simulink model "afe_abc_inv_psm_2mods"  (R2025a)
settings: Solver=ode1be  StartTime=0.0  StopTime=simlength  FixedStep=tc  MaxStep=tc
undefined symbols (not defined in the file): Ad_fht, Adrso, afe_pwm_phase_shift_mod1, afe_pwm_phase_shift_mod2, Amplitude_U, Amplitude_V, Amplitude_W, Aresd, b, Bresd, Cfht, Cresd, Crso, CTRPIFF_CLIP_RELEASE, dead_time_AFE, dead_time_INV, deepNEGeta, deepNEGxi, deepPOSxi, emf_fb_p, emf_fb_p_ccaller_1, emf_fb_p_ccaller_2, emf_p, emf_p_ccaller_1, emf_p_ccaller_2, enable_two_modules, end_time_LVRT, fPWM_AFE, fPWM_INV, g0_161Hz, g0_500Hz, g1_161Hz, g1_500Hz, i_grid_neg_eta_lim, i_grid_neg_eta_red_lim, i_grid_neg_xi_lim, i_grid_neg_xi_red_lim, i_grid_pos_eta_lim, i_grid_pos_eta_red_lim, ibez, id_lim, ieta_neg_ref_lim, ieta_pos_ref_lim, Igrid_phase_normalization_factor, inv_pwm_phase_shift_mod1, inv_pwm_phase_shift_mod2, iq_lim, ixi_pos_ref_lim, Jm, k_frt_ref, kg, ki_afe, ki_i, ki_rc_neg_grid, ki_rc_pos_grid, ki_vs, ki_w, kp_afe, kp_i, kp_rc_neg_grid ... (+64)
libraries: spsSampleandHoldLib x213, fl_lib x202, nesl_utility x126, simulink x22, cstblocks x18, threephase_inductor_lib x4, single_phase_transformer_lib x3, flexshaft_lib x1, pmsm_uvw_with_harmonics_lib x1
(part 17 of 18)

== system afe_abc_inv_psm_2mods/afe_abc_inv_psm_mod2/afe_control/grid_voltage_phase_lock_loops/DDSRF-PLL/pll_stageA/mormalization_and_transformation/Subsystem1 ==
  In : Inport
  Sample and Hold : spsSampleandHoldLib/Sample and Hold  ic=0  Ts=0
  Out : Outport
  wires:
  In/1 -> Sample and Hold/1
  [TRGO_afe_module_2] -> Sample and Hold/2
  Sample and Hold/1 -> Out/1

== system afe_abc_inv_psm_2mods/afe_abc_inv_psm_mod2/afe_control/grid_voltage_phase_lock_loops/DDSRF-PLL/pll_stageA/mormalization_and_transformation/Subsystem2 ==
  In : Inport
  Sample and Hold : spsSampleandHoldLib/Sample and Hold  ic=0  Ts=0
  Out : Outport
  wires:
  Sample and Hold/1 -> Out/1
  [TRGO_afe_module_2] -> Sample and Hold/2
  In/1 -> Sample and Hold/1

== system afe_abc_inv_psm_2mods/afe_abc_inv_psm_mod2/afe_control/grid_voltage_phase_lock_loops/DDSRF-PLL/pll_stageA/mormalization_and_transformation/Subsystem5 ==
  In : Inport
  Sample and Hold : spsSampleandHoldLib/Sample and Hold  ic=0  Ts=0
  Out : Outport
  wires:
  In/1 -> Sample and Hold/1
  [TRGO_afe_module_2] -> Sample and Hold/2
  Sample and Hold/1 -> Out/1

== system afe_abc_inv_psm_2mods/afe_abc_inv_psm_mod2/afe_control/grid_voltage_phase_lock_loops/DDSRF-PLL/pll_stageA/sequences/ddsrf ==
  u_grid_alpha : Inport
  u_grid_beta : Inport  Port=2
  phase_angle : Inport  Port=3
  Gain : Gain  Gain=2
  LTI System{,1..3} (4 alike) : cstblocks/LTI System  sys=ddsrf_fd  IC=[]  PadeOrder=0
  Sum : Sum  Inputs=|+-
  Sum1 : Sum  Inputs=|+-
  Sum2 : Sum  Inputs=-+|
  Sum3 : Sum  Inputs=-+|
  alphabeta2xieta_neg : MATLAB Function  TreatAsAtomicUnit=on
  alphabeta2xieta_neg1 : MATLAB Function  TreatAsAtomicUnit=on
  alphabeta2xieta_pos : MATLAB Function  TreatAsAtomicUnit=on
  alphabeta2xieta_pos1 : MATLAB Function  TreatAsAtomicUnit=on
  bounder2 : MATLAB Function  TreatAsAtomicUnit=on  SystemSampleTime=ts_afe
  u_grid_pos_xi : Outport
  u_grid_pos_eta : Outport  Port=2
  u_grid_neg_xi : Outport  Port=3
  u_grid_neg_eta : Outport  Port=4
  wires:
  alphabeta2xieta_neg1/2(eta) -> Sum3/1
  alphabeta2xieta_neg1/1(xi) -> Sum2/1
  alphabeta2xieta_pos1/2(eta) -> Sum1/2
  alphabeta2xieta_pos1/1(xi) -> Sum/2
  [phase_angle_2] -> alphabeta2xieta_neg1/3(gamma)
  [phase_angle_2] -> alphabeta2xieta_pos1/3(gamma)
  bounder2/1(y) -> [phase_angle_2]
  LTI System3/1 -> alphabeta2xieta_pos1/2(beta), u_grid_neg_eta/1
  LTI System2/1 -> alphabeta2xieta_pos1/1(alpha), u_grid_neg_xi/1
  LTI System1/1 -> u_grid_pos_eta/1, alphabeta2xieta_neg1/2(beta)
  LTI System/1 -> u_grid_pos_xi/1, alphabeta2xieta_neg1/1(alpha)
  Gain/1 -> bounder2/1(u)
  alphabeta2xieta_neg/2(eta) -> Sum3/2  "u_grid_neg_eta"
  Sum3/1 -> LTI System3/1
  Sum2/1 -> LTI System2/1
  alphabeta2xieta_neg/1(xi) -> Sum2/2  "u_grid_neg_xi"
  Sum1/1 -> LTI System1/1
  alphabeta2xieta_pos/2(eta) -> Sum1/1  "u_grid_pos_eta"
  Sum/1 -> LTI System/1
  alphabeta2xieta_pos/1(xi) -> Sum/1  "u_grid_pos_xi"
  u_grid_alpha/1 -> alphabeta2xieta_neg/1(alpha), alphabeta2xieta_pos/1(alpha)  "u_grid_alpha"
  u_grid_beta/1 -> alphabeta2xieta_neg/2(beta), alphabeta2xieta_pos/2(beta)  "u_grid_beta"
  phase_angle/1 -> Gain/1, alphabeta2xieta_neg/3(gamma), alphabeta2xieta_pos/3(gamma)  "phase_angle"

== system afe_abc_inv_psm_2mods/afe_abc_inv_psm_mod2/afe_control/grid_voltage_phase_lock_loops/DDSRF-PLL/pll_stageB/double_integrator_observer/Subsystem5 ==
  In : Inport
  Sample and Hold : spsSampleandHoldLib/Sample and Hold  ic=0  Ts=0
  Out : Outport
  wires:
  Sample and Hold/1 -> Out/1
  [TRGO_afe_module_1] -> Sample and Hold/2
  In/1 -> Sample and Hold/1

== system afe_abc_inv_psm_2mods/afe_abc_inv_psm_mod2/afe_control/grid_voltage_phase_lock_loops/DQ-PLL/pll_stageA/mormalization_and_transformation/Subsystem1 ==
  In : Inport
  Sample and Hold : spsSampleandHoldLib/Sample and Hold  ic=0  Ts=0
  Out : Outport
  wires:
  In/1 -> Sample and Hold/1
  [TRGO_afe_module_2] -> Sample and Hold/2
  Sample and Hold/1 -> Out/1

== system afe_abc_inv_psm_2mods/afe_abc_inv_psm_mod2/afe_control/grid_voltage_phase_lock_loops/DQ-PLL/pll_stageA/mormalization_and_transformation/Subsystem2 ==
  In : Inport
  Sample and Hold : spsSampleandHoldLib/Sample and Hold  ic=0  Ts=0
  Out : Outport
  wires:
  Sample and Hold/1 -> Out/1
  [TRGO_afe_module_2] -> Sample and Hold/2
  In/1 -> Sample and Hold/1

== system afe_abc_inv_psm_2mods/afe_abc_inv_psm_mod2/afe_control/grid_voltage_phase_lock_loops/DQ-PLL/pll_stageA/mormalization_and_transformation/Subsystem5 ==
  In : Inport
  Sample and Hold : spsSampleandHoldLib/Sample and Hold  ic=0  Ts=0
  Out : Outport
  wires:
  In/1 -> Sample and Hold/1
  [TRGO_afe_module_2] -> Sample and Hold/2
  Sample and Hold/1 -> Out/1

== system afe_abc_inv_psm_2mods/afe_abc_inv_psm_mod2/afe_control/grid_voltage_phase_lock_loops/DQ-PLL/pll_stageA/mormalization_and_transformation/u_500Hz_flt ==
  input : Inport
  Gain3 : Gain  Gain=g1_500Hz
  Gain6 : Gain  Gain=g0_500Hz
  Sum : Sum  Inputs=|++
  Unit Delay1 : UnitDelay  SampleTime=ts_afe  HasFrameUpgradeWarning=on
  output : Outport  VectorParamsAs1DForOutWhenUnconnected=off
  wires:
  Gain6/1 -> Sum/1
  input/1 -> Gain6/1
  Unit Delay1/1 -> Gain3/1
  Gain3/1 -> Sum/2
  Sum/1 -> Unit Delay1/1, output/1

== system afe_abc_inv_psm_2mods/afe_abc_inv_psm_mod2/afe_control/grid_voltage_phase_lock_loops/DQ-PLL/pll_stageA/mormalization_and_transformation/u_500Hz_flt1 ==
  input : Inport
  Gain3 : Gain  Gain=g1_500Hz
  Gain6 : Gain  Gain=g0_500Hz
  Sum : Sum  Inputs=|++
  Unit Delay1 : UnitDelay  SampleTime=ts_afe  HasFrameUpgradeWarning=on
  output : Outport  VectorParamsAs1DForOutWhenUnconnected=off
  wires:
  Sum/1 -> output/1, Unit Delay1/1
  Gain3/1 -> Sum/2
  Unit Delay1/1 -> Gain3/1
  input/1 -> Gain6/1
  Gain6/1 -> Sum/1

== system afe_abc_inv_psm_2mods/afe_abc_inv_psm_mod2/afe_control/grid_voltage_phase_lock_loops/DQ-PLL/pll_stageA/mormalization_and_transformation/u_500Hz_flt2 ==
  input : Inport
  Gain3 : Gain  Gain=g1_500Hz
  Gain6 : Gain  Gain=g0_500Hz
  Sum : Sum  Inputs=|++
  Unit Delay1 : UnitDelay  SampleTime=ts_afe  HasFrameUpgradeWarning=on
  output : Outport  VectorParamsAs1DForOutWhenUnconnected=off
  wires:
  Gain6/1 -> Sum/1
  input/1 -> Gain6/1
  Unit Delay1/1 -> Gain3/1
  Gain3/1 -> Sum/2
  Sum/1 -> Unit Delay1/1, output/1

== system afe_abc_inv_psm_2mods/afe_abc_inv_psm_mod2/afe_control/grid_voltage_phase_lock_loops/DQ-PLL/pll_stageA/sequences/alphabeta2xieta ==
  alpha : Inport
  beta : Inport  Port=2
  gamma : Inport  Port=3
  alphabeta2xieta_neg : MATLAB Function  TreatAsAtomicUnit=on  SystemSampleTime=ts_afe
  alphabeta2xieta_pos : MATLAB Function  TreatAsAtomicUnit=on  SystemSampleTime=ts_afe
  xi : Outport
  eta : Outport  Port=2
  Out3 : Outport  Port=3
  Out4 : Outport  Port=4
  wires:
  alphabeta2xieta_neg/2(eta) -> Out4/1  "u_grid_neg_eta"
  alphabeta2xieta_neg/1(xi) -> Out3/1  "u_grid_neg_xi"
  alphabeta2xieta_pos/2(eta) -> eta/1  "u_grid_pos_eta"
  alphabeta2xieta_pos/1(xi) -> xi/1  "u_grid_pos_xi"
  gamma/1 -> alphabeta2xieta_pos/3(gamma), alphabeta2xieta_neg/3(gamma)  "gamma_grid"
  beta/1 -> alphabeta2xieta_pos/2(beta), alphabeta2xieta_neg/2(beta)  "u_grid_beta"
  alpha/1 -> alphabeta2xieta_pos/1(alpha), alphabeta2xieta_neg/1(alpha)  "u_grid_alpha"

== system afe_abc_inv_psm_2mods/afe_abc_inv_psm_mod2/afe_control/grid_voltage_phase_lock_loops/DQ-PLL/pll_stageB/double_integrator_observer/Subsystem6 ==
  In : Inport
  Sample and Hold : spsSampleandHoldLib/Sample and Hold  ic=0  Ts=0
  Out : Outport
  wires:
  Sample and Hold/1 -> Out/1
  [TRGO_afe_module_1] -> Sample and Hold/2
  In/1 -> Sample and Hold/1

== system afe_abc_inv_psm_2mods/afe_abc_inv_psm_mod2/inverter_control/current_ctrl/bemf_observer/phase_fault/phase_fault/drop_phase_zerofor_delta_time ==
  theta_pmsm : Inport
  Product : Product
  Step : Step  Time=time_phase_fault  Before=1  After=0  SampleTime=0
  Step1 : Step  Time=time_phase_fault+3e-3  SampleTime=0
  Sum : Sum  Inputs=|++
  theta : Outport
  wires:
  Step/1 -> Sum/1
  Sum/1 -> Product/2
  Product/1 -> theta/1
  Step1/1 -> Sum/2
  theta_pmsm/1 -> Product/1

== system afe_abc_inv_psm_2mods/afe_abc_inv_psm_mod2/inverter_control/current_ctrl/bemf_observer/phase_fault/phase_fault/hold_phase_for_delta_time ==
  theta_pmsm : Inport
  Enabled Subsystem : Subsystem  TreatAsAtomicUnit=on
  Step : Step  Time=time_phase_fault  Before=1  After=0  SampleTime=0
  Step1 : Step  Time=time_phase_fault+25e-3  SampleTime=0
  Sum : Sum  Inputs=|++
  theta : Outport
  wires:
  Sum/1 -> Enabled Subsystem/Enable
  Enabled Subsystem/1(theta) -> theta/1
  theta_pmsm/1 -> Enabled Subsystem/1(theta_pmsm)
  Step1/1 -> Sum/2
  Step/1 -> Sum/1

== system afe_abc_inv_psm_2mods/afe_abc_inv_psm_mod2/inverter_control/current_ctrl/bemf_observer/phase_fault/phase_fault/loss_phase ==
  theta_pmsm : Inport
  Enabled Subsystem : Subsystem  TreatAsAtomicUnit=on
  Step : Step  Time=time_phase_fault  Before=1  After=0  SampleTime=0
  theta : Outport
  wires:
  theta_pmsm/1 -> Enabled Subsystem/1(theta_pmsm)
  Enabled Subsystem/1(theta) -> theta/1
  Step/1 -> Enabled Subsystem/Enable

== system afe_abc_inv_psm_2mods/afe_abc_inv_psm_mod2/inverter_control/current_ctrl/current_ctrl/dq_pi_with_vector_antiwindup/dq_vector_pi/bounder1 ==
  md : Inport
  m_1 : Inport  Port=2
  m : Inport  Port=3
  Constant : Constant
  Constant1 : Constant  Value=0
  Divide : Product
  Switch : Switch  Threshold=1  SaturateOnIntegerOverflow=off  InputSameDT=off
  Switch1 : Switch  Threshold=1  SaturateOnIntegerOverflow=off  InputSameDT=off
  md_sat : Outport  VectorParamsAs1DForOutWhenUnconnected=off
  clip : Outport  Port=2  VectorParamsAs1DForOutWhenUnconnected=off
  wires:
  Constant1/1 -> Switch/3
  Constant/1 -> Switch/1
  m/1 -> Switch/2, Switch1/2
  Switch/1 -> clip/1
  Switch1/1 -> md_sat/1
  Divide/1 -> Switch1/1
  m_1/1 -> Divide/1
  md/1 -> Divide/2, Switch1/3

== system afe_abc_inv_psm_2mods/afe_abc_inv_psm_mod2/inverter_control/current_ctrl/current_ctrl/dq_pi_with_vector_antiwindup/dq_vector_pi/bounder2 ==
  m : Inport
  m_1 : Inport  Port=2
  mq : Inport  Port=3
  Constant : Constant
  Constant1 : Constant  Value=0
  Divide : Product
  Switch : Switch  Threshold=1  SaturateOnIntegerOverflow=off  InputSameDT=off
  Switch1 : Switch  Threshold=1  SaturateOnIntegerOverflow=off  InputSameDT=off
  mq_sat : Outport  VectorParamsAs1DForOutWhenUnconnected=off
  clip : Outport  Port=2  VectorParamsAs1DForOutWhenUnconnected=off
  wires:
  mq/1 -> Switch1/3, Divide/2
  m_1/1 -> Divide/1
  Divide/1 -> Switch1/1
  Switch1/1 -> mq_sat/1
  Switch/1 -> clip/1
  m/1 -> Switch/2, Switch1/2
  Constant/1 -> Switch/1
  Constant1/1 -> Switch/3

== system afe_abc_inv_psm_2mods/afe_abc_inv_psm_mod2/inverter_control/current_ctrl/current_ctrl/dq_pi_with_vector_antiwindup/dq_vector_pi/pi_d ==
  id_tilde : Inport
  clip : Inport  Port=2
  1/Ti : Gain  Gain=kp_i  SaturateOnIntegerOverflow=on  OutDataTypeStr=Inherit: Same as input  ParamDataTypeStr=Inherit: Same as input
  Constant : Constant  Value=0
  Sum2 : Sum  Inputs=+-  SaturateOnIntegerOverflow=on
  Sum4 : Sum  SaturateOnIntegerOverflow=on
  Sum5 : Sum  SaturateOnIntegerOverflow=on
  Switch1 : Switch  Threshold=0.5  SaturateOnIntegerOverflow=off  InputSameDT=off
  Switch2 : Switch  Threshold=0.5  SaturateOnIntegerOverflow=off  InputSameDT=off
  Unit Delay1 : UnitDelay  SampleTime=ts_inv  HasFrameUpgradeWarning=on
  Unit Delay2 : UnitDelay  SampleTime=ts_inv  HasFrameUpgradeWarning=on
  kp1 : Gain  Gain=CTRPIFF_CLIP_RELEASE*ts_inv  SaturateOnIntegerOverflow=on  OutDataTypeStr=Inherit: Same as input  ParamDataTypeStr=Inherit: Same as input
  kp2 : Gain  Gain=ki_i*ts_inv  SaturateOnIntegerOverflow=on  OutDataTypeStr=Inherit: Same as input  ParamDataTypeStr=Inherit: Same as input
  ud_out : Outport  VectorParamsAs1DForOutWhenUnconnected=off
  wires:
  Unit Delay1/1 -> [clip]
  Constant/1 -> Switch2/1
  [clip] -> Switch1/2
  [clip] -> Switch2/2
  clip/1 -> Unit Delay1/1
  kp2/1 -> Switch2/3
  Switch2/1 -> Sum4/1
  1/Ti/1 -> Sum5/1
  Unit Delay2/1 -> Sum2/1, kp1/1, Sum4/2
  Sum2/1 -> Switch1/1
  kp1/1 -> Sum2/2
  Sum4/1 -> Switch1/3, Sum5/2
  Switch1/1 -> Unit Delay2/1
  Sum5/1 -> ud_out/1
  id_tilde/1 -> kp2/1, 1/Ti/1

== system afe_abc_inv_psm_2mods/afe_abc_inv_psm_mod2/inverter_control/current_ctrl/current_ctrl/dq_pi_with_vector_antiwindup/dq_vector_pi/pi_q ==
  iq_tilde : Inport
  clip : Inport  Port=2
  1/Ti : Gain  Gain=kp_i  SaturateOnIntegerOverflow=on  OutDataTypeStr=Inherit: Same as input  ParamDataTypeStr=Inherit: Same as input
  Constant : Constant  Value=0
  Sum2 : Sum  Inputs=+-  SaturateOnIntegerOverflow=on
  Sum4 : Sum  SaturateOnIntegerOverflow=on
  Sum5 : Sum  SaturateOnIntegerOverflow=on
  Switch1 : Switch  Threshold=0.5  SaturateOnIntegerOverflow=off  InputSameDT=off
  Switch2 : Switch  Threshold=0.5  SaturateOnIntegerOverflow=off  InputSameDT=off
  Unit Delay1 : UnitDelay  SampleTime=ts_inv  HasFrameUpgradeWarning=on
  Unit Delay2 : UnitDelay  SampleTime=ts_inv  HasFrameUpgradeWarning=on
  kp1 : Gain  Gain=CTRPIFF_CLIP_RELEASE*ts_inv  SaturateOnIntegerOverflow=on  OutDataTypeStr=Inherit: Same as input  ParamDataTypeStr=Inherit: Same as input
  kp2 : Gain  Gain=ki_i*ts_inv  SaturateOnIntegerOverflow=on  OutDataTypeStr=Inherit: Same as input  ParamDataTypeStr=Inherit: Same as input
  Vqs_out : Outport  VectorParamsAs1DForOutWhenUnconnected=off
  wires:
  Sum5/1 -> Vqs_out/1
  Unit Delay1/1 -> [clip]
  iq_tilde/1 -> kp2/1, 1/Ti/1
  Switch1/1 -> Unit Delay2/1
  Sum4/1 -> Switch1/3, Sum5/2
  kp1/1 -> Sum2/2
  Sum2/1 -> Switch1/1
  Unit Delay2/1 -> Sum4/2, kp1/1, Sum2/1
  1/Ti/1 -> Sum5/1
  Switch2/1 -> Sum4/1
  kp2/1 -> Switch2/3
  clip/1 -> Unit Delay1/1
  [clip] -> Switch2/2
  [clip] -> Switch1/2
  Constant/1 -> Switch2/1

== system afe_abc_inv_psm_2mods/afe_abc_inv_psm_mod2/inverter_control/current_ctrl/current_ctrl/dq_pi_with_vector_antiwindup/dq_vector_pi/switch ==
  clip 1 : Inport
  clip 2 : Inport  Port=2
  Constant4 : Constant
  Constant5 : Constant  Value=0
  Sum1 : Sum  SaturateOnIntegerOverflow=on
  Switch : Switch  Threshold=0.5  SaturateOnIntegerOverflow=off  InputSameDT=off
  clip : Outport  VectorParamsAs1DForOutWhenUnconnected=off
  wires:
  clip 2/1 -> Sum1/2
  clip 1/1 -> Sum1/1
  Sum1/1 -> Switch/2
  Constant4/1 -> Switch/1
  Switch/1 -> clip/1
  Constant5/1 -> Switch/3

== system afe_abc_inv_psm_2mods/afe_abc_inv_psm_mod2/inverter_control/current_ctrl/current_ctrl/dq_pi_with_vector_antiwindup/dq_vector_pi/vector lenght ==
  md : Inport
  mq : Inport  Port=2
  Math Function : Math  Operator=magnitude^2  SignedPower=on
  Math Function1 : Math  Operator=magnitude^2  SignedPower=on
  Math Function2 : Math  Operator=reciprocal  SignedPower=on
  Sqrt : Sqrt
  Sum5 : Sum  SaturateOnIntegerOverflow=on
  m_1 : Outport  VectorParamsAs1DForOutWhenUnconnected=off
  m : Outport  Port=2  VectorParamsAs1DForOutWhenUnconnected=off
  wires:
  md/1 -> Math Function/1
  Math Function2/1 -> m_1/1
  Sum5/1 -> Sqrt/1
  Math Function/1 -> Sum5/1
  Math Function1/1 -> Sum5/2
  mq/1 -> Math Function1/1
  Sqrt/1 -> Math Function2/1, m/1

== system afe_abc_inv_psm_2mods/afe_abc_inv_psm_mod2/inverter_control/current_ctrl/current_ctrl/dq_pi_with_vector_antiwindup/dq_vector_pi_ccaller/Reset ==
  Step : Step  Time=0.05  Before=1  After=0  SampleTime=0
  en : Outport
  wires:
  Step/1 -> en/1

== system afe_abc_inv_psm_2mods/afe_abc_inv_psm_mod2/inverter_control/current_ctrl/current_ctrl/dq_pi_with_vector_antiwindup/dq_vector_pi_ccaller/Subsystem1 ==
  In : Inport
  Sample and Hold : spsSampleandHoldLib/Sample and Hold  ic=0  Ts=0
  Out : Outport
  wires:
  Sample and Hold/1 -> Out/1
  [TRGO_inv_module_2] -> Sample and Hold/2
  In/1 -> Sample and Hold/1

== system afe_abc_inv_psm_2mods/afe_abc_inv_psm_mod2/inverter_control/current_ctrl/current_ctrl/dq_pi_with_vector_antiwindup/dq_vector_pi_ccaller/Subsystem10 ==
  In : Inport
  Sample and Hold : spsSampleandHoldLib/Sample and Hold  ic=0  Ts=0
  Out : Outport
  wires:
  In/1 -> Sample and Hold/1
  [TRGO_inv_module_2] -> Sample and Hold/2
  Sample and Hold/1 -> Out/1

== system afe_abc_inv_psm_2mods/afe_abc_inv_psm_mod2/inverter_control/current_ctrl/current_ctrl/dq_pi_with_vector_antiwindup/dq_vector_pi_ccaller/Subsystem11 ==
  In : Inport
  Sample and Hold : spsSampleandHoldLib/Sample and Hold  ic=0  Ts=0
  Out : Outport
  wires:
  Sample and Hold/1 -> Out/1
  [TRGO_inv_module_2] -> Sample and Hold/2
  In/1 -> Sample and Hold/1

== system afe_abc_inv_psm_2mods/afe_abc_inv_psm_mod2/inverter_control/current_ctrl/current_ctrl/dq_pi_with_vector_antiwindup/dq_vector_pi_ccaller/Subsystem2 ==
  In : Inport
  Sample and Hold : spsSampleandHoldLib/Sample and Hold  ic=0  Ts=0
  Out : Outport
  wires:
  In/1 -> Sample and Hold/1
  [TRGO_inv_module_2] -> Sample and Hold/2
  Sample and Hold/1 -> Out/1

== system afe_abc_inv_psm_2mods/afe_abc_inv_psm_mod2/inverter_control/current_ctrl/current_ctrl/dq_pi_with_vector_antiwindup/dq_vector_pi_ccaller/Subsystem23 ==
  In : Inport
  Sample and Hold : spsSampleandHoldLib/Sample and Hold  ic=0  Ts=0
  Out : Outport
  wires:
  In/1 -> Sample and Hold/1
  [TRGO_inv_module_2] -> Sample and Hold/2
  Sample and Hold/1 -> Out/1

== system afe_abc_inv_psm_2mods/afe_abc_inv_psm_mod2/inverter_control/current_ctrl/current_ctrl/dq_pi_with_vector_antiwindup/dq_vector_pi_ccaller/Subsystem3 ==
  In : Inport
  Sample and Hold : spsSampleandHoldLib/Sample and Hold  ic=0  Ts=0
  Out : Outport
  wires:
  Sample and Hold/1 -> Out/1
  [TRGO_inv_module_2] -> Sample and Hold/2
  In/1 -> Sample and Hold/1

== system afe_abc_inv_psm_2mods/afe_abc_inv_psm_mod2/inverter_control/current_ctrl/current_ctrl/dq_pi_with_vector_antiwindup/dq_vector_pi_ccaller/Subsystem4 ==
  In : Inport
  Sample and Hold : spsSampleandHoldLib/Sample and Hold  ic=0  Ts=0
  Out : Outport
  wires:
  In/1 -> Sample and Hold/1
  [TRGO_inv_module_2] -> Sample and Hold/2
  Sample and Hold/1 -> Out/1

== system afe_abc_inv_psm_2mods/afe_abc_inv_psm_mod2/inverter_control/current_ctrl/current_ctrl/dq_pi_with_vector_antiwindup/dq_vector_pi_ccaller/Subsystem5 ==
  In : Inport
  Sample and Hold : spsSampleandHoldLib/Sample and Hold  ic=0  Ts=0
  Out : Outport
  wires:
  Sample and Hold/1 -> Out/1
  [TRGO_inv_module_2] -> Sample and Hold/2
  In/1 -> Sample and Hold/1

== system afe_abc_inv_psm_2mods/afe_abc_inv_psm_mod2/inverter_control/current_ctrl/current_ctrl/dq_pi_with_vector_antiwindup/dq_vector_pi_ccaller/Subsystem6 ==
  In : Inport
  Sample and Hold : spsSampleandHoldLib/Sample and Hold  ic=0  Ts=0
  Out : Outport
  wires:
  In/1 -> Sample and Hold/1
  [TRGO_inv_module_2] -> Sample and Hold/2
  Sample and Hold/1 -> Out/1

== system afe_abc_inv_psm_2mods/afe_abc_inv_psm_mod2/inverter_control/current_ctrl/current_ctrl/dq_pi_with_vector_antiwindup/dq_vector_pi_ccaller/Subsystem7 ==
  In : Inport
  Sample and Hold : spsSampleandHoldLib/Sample and Hold  ic=0  Ts=0
  Out : Outport
  wires:
  Sample and Hold/1 -> Out/1
  [TRGO_inv_module_2] -> Sample and Hold/2
  In/1 -> Sample and Hold/1

== system afe_abc_inv_psm_2mods/afe_abc_inv_psm_mod2/inverter_control/current_ctrl/current_ctrl/dq_pi_with_vector_antiwindup/dq_vector_pi_ccaller/Subsystem8 ==
  In : Inport
  Sample and Hold : spsSampleandHoldLib/Sample and Hold  ic=0  Ts=0
  Out : Outport
  wires:
  In/1 -> Sample and Hold/1
  [TRGO_inv_module_2] -> Sample and Hold/2
  Sample and Hold/1 -> Out/1

== system afe_abc_inv_psm_2mods/afe_abc_inv_psm_mod2/inverter_control/current_ctrl/current_ctrl/dq_pi_with_vector_antiwindup/dq_vector_pi_ccaller/Subsystem9 ==
  In : Inport
  Sample and Hold : spsSampleandHoldLib/Sample and Hold  ic=0  Ts=0
  Out : Outport
  wires:
  Sample and Hold/1 -> Out/1
  [TRGO_inv_module_2] -> Sample and Hold/2
  In/1 -> Sample and Hold/1

== system afe_abc_inv_psm_2mods/afe_abc_inv_psm_mod1/inverter_control/current_ctrl/bemf_observer/phase_fault/phase_fault/hold_phase_for_delta_time/Enabled Subsystem ==
  theta_pmsm : Inport
  Enable : EnablePort
  theta : Outport
  wires:
  theta_pmsm/1 -> theta/1

== system afe_abc_inv_psm_2mods/afe_abc_inv_psm_mod1/inverter_control/current_ctrl/bemf_observer/phase_fault/phase_fault/loss_phase/Enabled Subsystem ==
  theta_pmsm : Inport
  Enable : EnablePort
  theta : Outport
  wires:
  theta_pmsm/1 -> theta/1

== system afe_abc_inv_psm_2mods/afe_abc_inv_psm_mod2/inverter_control/current_ctrl/bemf_observer/phase_fault/phase_fault/hold_phase_for_delta_time/Enabled Subsystem ==
  theta_pmsm : Inport
  Enable : EnablePort
  theta : Outport
  wires:
  theta_pmsm/1 -> theta/1

== system afe_abc_inv_psm_2mods/afe_abc_inv_psm_mod2/inverter_control/current_ctrl/bemf_observer/phase_fault/phase_fault/loss_phase/Enabled Subsystem ==
  theta_pmsm : Inport
  Enable : EnablePort
  theta : Outport
  wires:
  theta_pmsm/1 -> theta/1

== matlab function afe_abc_inv_psm_2mods/afe_abc_inv_psm_mod1/afe_control/current_ctrl/current_transformation/alphabeta2xieta ==
  data: alpha input; xi output; beta input; gamma input; eta output
function [xi,eta] = alphabeta2xieta(alpha,beta,gamma)

    xi  =  alpha*cos(gamma) + beta*sin(gamma);
    eta = -alpha*sin(gamma) + beta*cos(gamma);

end

== matlab function afe_abc_inv_psm_2mods/grid/grid_emulator/grid_emulator/voltage_reference/xieta2alphabeta_pos ==
  data: xi input; alpha output; eta input; gamma input; beta output
function [alpha,beta] = xieta2alphabeta_pos(xi,eta,gamma)

    alpha  =  xi*cos(gamma) - eta*sin(gamma);
    beta = xi*sin(gamma) + eta*cos(gamma);

end

== matlab function afe_abc_inv_psm_2mods/afe_abc_inv_psm_mod1/inverter_control/current_ctrl/current_transformation/uvw2alphabeta ==
  data: u input; alpha output; v input; w input; beta output
function [alpha,beta] = uvw2alphabeta(u,v,w)

alpha = 2/3*(u - 1/2*v - 1/2*w);
beta  = 2/3*(sqrt(3)/2*(v - w));

end

== matlab function afe_abc_inv_psm_2mods/afe_abc_inv_psm_mod1/inverter_control/current_ctrl/dq2alphabeta ==
  data: d input; alpha output; q input; gamma input; beta output
function [alpha,beta] = dq2alphabeta(d,q,gamma)

    alpha  =  d*cos(gamma) - q*sin(gamma);
    beta = d*sin(gamma) + q*cos(gamma);

end

== matlab function afe_abc_inv_psm_2mods/afe_abc_inv_psm_mod1/afe_control/FRT-VDE4110/FRT-Detection/LVRT_detector ==
  data: vxi_p input; vxi_n input; veta_n input; vxi_p_dot input; vxi_n_dot input; enable input; red_dyn_enabled input; pwr_lim_enable output; frt_exceeded output; reset input; frt_active output; frt_state output; red_dyn_active output
function [pwr_lim_enable, frt_exceeded, frt_active, frt_state, red_dyn_active]  = lvrt_detector(vxi_p,vxi_n,veta_n,vxi_p_dot,vxi_n_dot, enable, red_dyn_enabled, reset)

    persistent state count count2 state_pwr_lim
    
    LVRT_IDLE = 0;
    LVRT_ACTIVE = 1;
    LVRT_EXCEEDED = 2;
    
    PWR_LIM_DISABLED = 0;
    PWR_LIM_ENABLED  = 1;
    
    LVRT_VPOS_TH_LOW			= 0.85;
    LVRT_VPOS_TH_HIGH			= 1.15;
    LVRT_SEQ_DETECTION_HYST		= 0.1;
    LVRT_VNEG_TH				= 0.1;
    LVRT_VPOS_DOT_TH			= 3.0;
    LVRT_VNEG_DOT_TH			= 3.0;
    LVRT_VPOS_PWRLIM_TH			= 0.8;
    LVRT_VNEG_PWRLIM_TH			= 0.1;
    LVRT_PWRLIM_HYST			= 0.1;
    LVRT_VPOS_RED_DYN_TH        = 0.7;
    LVRT_VNEG_RED_DYN_TH        = 0.2;
    LVRT_TIME_HOLD_MAX          = 61000;
    
    RED_DYN_NOT_ACTIVE = 0;
    RED_DYN_ACTIVE     = 1;
        
    if isempty(state)
        state = LVRT_IDLE;
        state_pwr_lim = PWR_LIM_DISABLED;
        count = 0;
        count2 = 0;
    end

    vn = sqrt(vxi_n^2+veta_n^2);

    if enable == 1
        
        switch state
            
            case LVRT_IDLE
                if ((vxi_p > LVRT_VPOS_TH_HIGH || vxi_p < LVRT_VPOS_TH_LOW || vn > LVRT_VNEG_TH) ...
                     && (vxi_p_dot > LVRT_VPOS_DOT_TH || vxi_n_dot > LVRT_VNEG_DOT_TH) && ...
                     count2 > 1000)
                    state = LVRT_ACTIVE;
                end
                frt_active = 0;
                frt_exceeded = 0;
                count = 0;
                frt_state = LVRT_IDLE;
                state_pwr_lim = PWR_LIM_DISABLED;                  
                red_dyn_active = RED_DYN_NOT_ACTIVE;
                count2 = count2 + 1;

            case LVRT_ACTIVE
                count2 = 0;
                % LVRT condition not active anymore
                if (vxi_p >= LVRT_VPOS_TH_LOW  + LVRT_SEQ_DETECTION_HYST && ...
                    vxi_p <  LVRT_VPOS_TH_HIGH - LVRT_SEQ_DETECTION_HYST)
                    state = LVRT_IDLE;
                % LVRT exceeded
                elseif (count >= LVRT_TIME_HOLD_MAX)
                    state = LVRT_EXCEEDED;
                end
                
                % handle power limitation
                if (vxi_p < LVRT_VPOS_PWRLIM_TH || vn > LVRT_VNEG_PWRLIM_TH) 
                    state_pwr_lim = PWR_LIM_ENABLED;
                elseif (vxi_p > LVRT_VPOS_PWRLIM_TH + LVRT_PWRLIM_HYST && vn < LVRT_VPOS_PWRLIM_TH - LVRT_PWRLIM_HYST)
                    state_pwr_lim = PWR_LIM_DISABLED;                  
                end
                
                % handle reduced dynamic grid support
                if red_dyn_enabled && (vxi_p < LVRT_VPOS_RED_DYN_TH || vn > LVRT_VNEG_RED_DYN_TH)
                    red_dyn_active = RED_DYN_ACTIVE;
                else
                    red_dyn_active = RED_DYN_NOT_ACTIVE;
                end
                 
                frt_active = 1;
                frt_exceeded = 0;
                frt_state = LVRT_ACTIVE;
                
                count = count + 1;
            
            case LVRT_EXCEEDED

                if ((reset == 1) || (enable == 0))
                    state = LVRT_IDLE;
                else
                    state = LVRT_EXCEEDED;
                end
                
                frt_exceeded = 1;
                frt_active = 0; 
                frt_state = LVRT_EXCEEDED;
                red_dyn_active = RED_DYN_NOT_ACTIVE;
            
            otherwise
                state = LVRT_IDLE;
                frt_active = 0;
                frt_exceeded = 0;
                frt_state = LVRT_IDLE;
                red_dyn_active = RED_DYN_NOT_ACTIVE;
        end
        
        if state_pwr_lim == PWR_LIM_ENABLED
            pwr_lim_enable = 1;
        else
            pwr_lim_enable = 0;
        end      
    else
        state = LVRT_IDLE;
        frt_active = 0;
        pwr_lim_enable = 0;
        frt_exceeded = 0;
        frt_state = LVRT_IDLE;
        red_dyn_active = RED_DYN_NOT_ACTIVE;
    end
end

== matlab function afe_abc_inv_psm_2mods/afe_abc_inv_psm_mod1/brake/MATLAB Function ==
  data: u input; y output; udc_ref input
function y = fcn(u,udc_ref)

persistent enable_brake

udc_brake_min = 1.15;
udc_brake_max = 1.175;

if isempty(enable_brake)
    enable_brake = 0
end

if u >= udc_ref*udc_brake_max
    y = 15;
    enable_brake = 1;
elseif (u < udc_ref*udc_brake_max && u >= udc_ref*udc_brake_min && enable_brake == 1)
    y = 15;
    enable_brake = 1;
elseif (u < udc_ref*udc_brake_max && u >= udc_ref*udc_brake_min && enable_brake == 0)
    y = 0;
    enable_brake = 0;
else
    y = 0;
    enable_brake = 0;
end

% function y = fcn(u,udc_ref)
% 
% persistent enable_brake
% 
% udc_brake_min = 1.145;
% udc_brake_max = 1.165;
% 
% if isempty(enable_brake)
%     enable_brake = 0
% end
% 
% if u >= udc_ref*udc_brake_max
%     y = 15;
%     enable_brake = 1;
% elseif (u < udc_ref*udc_brake_max && u >= udc_ref*udc_brake_min && enable_brake == 1)
%     y = 15;
%     enable_brake = 1;
% elseif (u < udc_ref*udc_brake_max && u >= udc_ref*udc_brake_min && enable_brake == 0)
%     y = 0;
%     enable_brake = 0;
% else
%     y = 0;
%     enable_brake = 0;
end

== matlab function afe_abc_inv_psm_2mods/afe_abc_inv_psm_mod1/inverter/inverter/sv_pwm/modulator1/PWM generator 2/MATLAB Function ==
  data: t input; y output; phase input; period input
function y = trgo(t,phase,period)
x = sin(2*pi/period*t - phase -pi/2);
y = asin(x);

== matlab function afe_abc_inv_psm_2mods/afe_abc_inv_psm_mod1/afe/sv_pwm/modulator1/PWM generator 3/MATLAB Function ==
  data: t input; y output; phase input; period input
function y = trgo(t,phase,period)
x = sin(2*pi/period*t - phase -pi/2);
y = asin(x);

== matlab function afe_abc_inv_psm_2mods/afe_abc_inv_psm_mod1/inverter_control/current_ctrl/bemf_observer/phase_fault/double_integrator_observer/bounder2 ==
  data: u input; y output
function y = bounder(u)
    
    u = -pi + mod(u+3*pi,2*pi);
    
    y = u;
end

== matlab function afe_abc_inv_psm_2mods/afe_abc_inv_psm_mod1/afe/sv_pwm/modulator1/PWM generator 1/MATLAB Function ==
  data: t input; y output; phase input; period input
function y = trgo(t,phase,period)
x = sin(2*pi/period*t - phase -pi/2);
y = asin(x);

== matlab function afe_abc_inv_psm_2mods/grid/grid_emulator/grid_emulator/voltage_reference/voltage_dource_with_frt/Phase_a1 ==
  data: A input; y output; phi input
function y = Phase_a(A,phi)

    y = A*cos(phi);

end

== matlab function afe_abc_inv_psm_2mods/grid/grid_emulator/grid_emulator/voltage_reference/voltage_dource_with_frt/Phase_b1 ==
  data: A input; y output; phi input
function y = Phase_b(A,phi)

    y = A*cos(phi-2*pi/3);

end

== matlab function afe_abc_inv_psm_2mods/grid/grid_emulator/grid_emulator/voltage_reference/voltage_dource_with_frt/Phase_c1 ==
  data: A input; y output; phi input
function y = Phase_c(A,phi)

    y = A*cos(phi-4*pi/3);

end

== matlab function afe_abc_inv_psm_2mods/afe_abc_inv_psm_mod1/inverter/inverter/sv_pwm/modulator1/PWM generator 3/MATLAB Function ==
  data: t input; y output; phase input; period input
function y = trgo(t,phase,period)
x = sin(2*pi/period*t - phase -pi/2);
y = asin(x);

== matlab function afe_abc_inv_psm_2mods/afe_abc_inv_psm_mod1/inverter_control/current_ctrl/bemf_observer/bemf_observer/double_integrator_observer/bounder1 ==
  data: u input; y output
function y = bounder(u)
    
    y = -pi + mod(u+3*pi,2*pi);
end

== matlab function afe_abc_inv_psm_2mods/afe_abc_inv_psm_mod1/inverter_control/current_ctrl/bemf_observer/bemf_observer/double_integrator_observer/bounder2 ==
  data: u input; y output
function y = bounder(u)
    
    u = -pi + mod(u+3*pi,2*pi);
    
    y = u;
end

== matlab function afe_abc_inv_psm_2mods/afe_abc_inv_psm_mod1/afe_control/FRT-VDE4110/FRT-PosNegReactiveCurrentReferences/avg_flt_500ms/avg_flt_1 ==
  data: x input; y1 output; w input; ts input; enable input
function y1  = avg_flt(x,w,ts, enable)

    persistent x_int x_int_1 y_N N

    N = (1/(w/(2*pi)))/ts+1;

    if isempty(x_int)
        x_int_1 = 0;
        y_N = zeros(1,N);
        y1 = 0;
    end


    if enable == 1
        x_int = x * ts * w + x_int_1;
        x_int_1 = x_int;
        y_N(1,1) = x_int;
        y1 = 1/(2*pi)*((y_N(1,1) - y_N(1,N)));
        for i = 1:(N-1)
            y_N(1,N+1-i) = y_N(1,N-i); 
        end
    else
        y1 = 1/(2*pi)*((y_N(1,1) - y_N(1,N)));
    end
end

== matlab function afe_abc_inv_psm_2mods/afe_abc_inv_psm_mod1/afe_control/grid_voltage_phase_lock_loops/dq_pll/pll_stageA/mormalization_and_transformation/abc2alphabeta ==
  data: a input; alpha output; b input; c input; beta output
function [alpha,beta] = abc2alphabeta(a,b,c)

alpha = 2/3*(a - 1/2*b - 1/2*c);
beta  = 1/sqrt(3)*(b - c);

end

== matlab function afe_abc_inv_psm_2mods/afe_abc_inv_psm_mod1/afe_control/grid_voltage_phase_lock_loops/dq_pll/pll_stageA/sequences/alphabeta2xieta/alphabeta2xieta_neg ==
  data: alpha input; xi output; beta input; gamma input; eta output
function [xi,eta] = alphabeta2xieta_neg(alpha,beta,gamma)

    xi  = alpha*cos(gamma) - beta*sin(gamma);
    eta = alpha*sin(gamma) + beta*cos(gamma);

end

== matlab function afe_abc_inv_psm_2mods/afe_abc_inv_psm_mod1/afe_control/grid_voltage_phase_lock_loops/dq_pll/pll_stageA/sequences/alphabeta2xieta/alphabeta2xieta_pos ==
  data: alpha input; xi output; beta input; gamma input; eta output
function [xi,eta] = alphabeta2xieta_pos(alpha,beta,gamma)

    xi  =  alpha*cos(gamma) + beta*sin(gamma);
    eta = -alpha*sin(gamma) + beta*cos(gamma);

end

== matlab function afe_abc_inv_psm_2mods/afe_abc_inv_psm_mod1/afe_control/grid_voltage_phase_lock_loops/dq_pll/pll_stageB/double_integrator_observer/bounder1 ==
  data: u input; y output
function y = bounder(u)
    
    u = -pi + mod(u+3*pi,2*pi);
    
    y = u;
end

== matlab function afe_abc_inv_psm_2mods/afe_abc_inv_psm_mod1/afe_control/grid_voltage_phase_lock_loops/dq_pll/pll_stageB/double_integrator_observer/bounder2 ==
  data: u input; y output
function y = bounder(u)
    
    u = -pi + mod(u+3*pi,2*pi);
    
    y = u;
end

== matlab function afe_abc_inv_psm_2mods/afe_abc_inv_psm_mod1/afe_control/grid_voltage_phase_lock_loops/dq_pll/pll_stageB/bounder1 ==
  data: u input; y output
function y = bounder(u)
    
    u = -pi + mod(u+3*pi,2*pi);
    
    y = u;
end

== matlab function afe_abc_inv_psm_2mods/grid/grid_emulator/grid_emulator/phase_gen/bounder1 ==
  data: u input; y output
function y = bounder(u)    
    y = -pi + mod(u+3*pi,2*pi);
end

== matlab function afe_abc_inv_psm_2mods/afe_abc_inv_psm_mod1/afe_control/FRT-VDE4110/FRT-PosNegReactiveCurrentReferences/avg_flt_500ms1/avg_flt_1 ==
  data: x input; y1 output; w input; ts input; enable input
function y1  = avg_flt(x,w,ts, enable)

    persistent x_int x_int_1 y_N N

    N = (1/(w/(2*pi)))/ts+1;

    if isempty(x_int)
        x_int_1 = 0;
        y_N = zeros(1,N);
        y1 = 0;
    end


    if enable == 1
        x_int = x * ts * w + x_int_1;
        x_int_1 = x_int;
        y_N(1,1) = x_int;
        y1 = 1/(2*pi)*((y_N(1,1) - y_N(1,N)));
        for i = 1:(N-1)
            y_N(1,N+1-i) = y_N(1,N-i); 
        end
    else
        y1 = 1/(2*pi)*((y_N(1,1) - y_N(1,N)));
    end
end

== matlab function afe_abc_inv_psm_2mods/afe_abc_inv_psm_mod1/afe_control/FRT-VDE4110/FRT-PosNegReactiveCurrentReferences/avg_flt_500ms2/avg_flt_1 ==
  data: x input; y1 output; w input; ts input; enable input
function y1  = avg_flt(x,w,ts, enable)

    persistent x_int x_int_1 y_N N

    N = (1/(w/(2*pi)))/ts+1;

    if isempty(x_int)
        x_int_1 = 0;
        y_N = zeros(1,N);
        y1 = 0;
    end


    if enable == 1
        x_int = x * ts * w + x_int_1;
        x_int_1 = x_int;
        y_N(1,1) = x_int;
        y1 = 1/(2*pi)*((y_N(1,1) - y_N(1,N)));
        for i = 1:(N-1)
            y_N(1,N+1-i) = y_N(1,N-i); 
        end
    else
        y1 = 1/(2*pi)*((y_N(1,1) - y_N(1,N)));
    end
end

== matlab function afe_abc_inv_psm_2mods/afe_abc_inv_psm_mod1/afe_control/FRT-VDE4110/FRT-PosNegReactiveCurrentReferences/avg_flt_500ms3/avg_flt_1 ==
  data: x input; y1 output; w input; ts input; enable input
function y1  = avg_flt(x,w,ts, enable)

    persistent x_int x_int_1 y_N N

    N = (1/(w/(2*pi)))/ts+1;

    if isempty(x_int)
        x_int_1 = 0;
        y_N = zeros(1,N);
        y1 = 0;
    end


    if enable == 1
        x_int = x * ts * w + x_int_1;
        x_int_1 = x_int;
        y_N(1,1) = x_int;
        y1 = 1/(2*pi)*((y_N(1,1) - y_N(1,N)));
        for i = 1:(N-1)
            y_N(1,N+1-i) = y_N(1,N-i); 
        end
    else
        y1 = 1/(2*pi)*((y_N(1,1) - y_N(1,N)));
    end
end

== matlab function afe_abc_inv_psm_2mods/afe_abc_inv_psm_mod1/afe_control/v_alphabeta2xieta/MATLAB Function ==
  data: alpha input; xi output; beta input; gamma input; eta output
function [xi,eta] = alphabeta2pos(alpha,beta,gamma)

    xi  =  alpha*cos(gamma) + beta*sin(gamma);
    eta = -alpha*sin(gamma) + beta*cos(gamma);

end

== matlab function afe_abc_inv_psm_2mods/afe_abc_inv_psm_mod1/afe_control/v_alphabeta2xieta/MATLAB Function1 ==
  data: alpha input; xi output; beta input; gamma input; eta output
function [xi,eta] = alphabeta2neg(alpha,beta,gamma)

    xi  = alpha*cos(gamma) - beta*sin(gamma);
    eta = alpha*sin(gamma) + beta*cos(gamma);

end

== matlab function afe_abc_inv_psm_2mods/afe_abc_inv_psm_mod1/afe_control/grid_voltage_sampling_and_alpha_beta_transformation/v_abc2alphabeta ==
  data: v_abc input; alpha output; beta output
function [alpha,beta] = abc2alphabeta(v_abc)

alpha = 2/3*(v_abc(1) - 1/2*v_abc(2) - 1/2*v_abc(3));
beta  = 1/sqrt(3)*(v_abc(2) - v_abc(3));

end

== matlab function afe_abc_inv_psm_2mods/afe_abc_inv_psm_mod1/afe_control/i_alphabeta2xieta/MATLAB Function ==
  data: alpha input; xi output; beta input; gamma input; eta output
function [xi,eta] = alphabeta2pos(alpha,beta,gamma)

    xi  =  alpha*cos(gamma) + beta*sin(gamma);
    eta = -alpha*sin(gamma) + beta*cos(gamma);

end

== matlab function afe_abc_inv_psm_2mods/afe_abc_inv_psm_mod1/afe_control/i_alphabeta2xieta/MATLAB Function1 ==
  data: alpha input; xi output; beta input; gamma input; eta output
function [xi,eta] = alphabeta2neg(alpha,beta,gamma)

    xi  = alpha*cos(gamma) - beta*sin(gamma);
    eta = alpha*sin(gamma) + beta*cos(gamma);

end

== matlab function afe_abc_inv_psm_2mods/afe_abc_inv_psm_mod1/afe_control/grid_current_sampling_and_alpha_beta_transformation/i_abc2alphabeta ==
  data: i_abc input; alpha output; beta output
function [alpha,beta] = abc2alphabeta(i_abc)

alpha = 2/3*(i_abc(1) - 1/2*i_abc(2) - 1/2*i_abc(3));
beta  = 1/sqrt(3)*(i_abc(2) - i_abc(3));

end

== matlab function afe_abc_inv_psm_2mods/afe_abc_inv_psm_mod1/afe_control/current_ctrl/Inner Loop Current Control/MATLAB Function ==
  data: a input; alpha output; b input; c input; beta output
function [alpha,beta] = abc2alphabeta(a,b,c)

alpha = 2/3*(a - 1/2*b - 1/2*c);
beta  = 1/sqrt(3)*(b - c);

end

== matlab function afe_abc_inv_psm_2mods/afe_abc_inv_psm_mod1/afe_control/current_ctrl/xieta2abc/MATLAB Function2 ==
  data: alpha input; a output; beta input; b output; c output
function [a,b,c] = alphabeta2abc(alpha,beta)

a = alpha;
b = -(1/2)*alpha + sqrt(3)/2*beta;
c = -(1/2)*alpha - sqrt(3)/2*beta;

end

== matlab function afe_abc_inv_psm_2mods/afe_abc_inv_psm_mod1/afe_control/current_ctrl/xieta2abc/Negative Sequence ==
  data: xi input; alpha output; eta input; gamma input; beta output
function [alpha,beta] = neg2alphabeta(xi,eta,gamma)

    alpha = xi*cos(gamma)  + eta*sin(gamma);
    beta  = -xi*sin(gamma) + eta*cos(gamma);

end

== matlab function afe_abc_inv_psm_2mods/afe_abc_inv_psm_mod1/afe_control/current_ctrl/xieta2abc/Positive Sequence ==
  data: xi input; alpha output; eta input; gamma input; beta output
function [alpha,beta] = pos2alphabeta(xi,eta,gamma)

    alpha = xi*cos(gamma) - eta*sin(gamma);
    beta  = xi*sin(gamma) + eta*cos(gamma);

end

== matlab function afe_abc_inv_psm_2mods/afe_abc_inv_psm_mod1/inverter/inverter/sv_pwm/modulator1/PWM generator 1/MATLAB Function ==
  data: t input; y output; phase input; period input
function y = trgo(t,phase,period)
x = sin(2*pi/period*t - phase -pi/2);
y = asin(x);

== matlab function afe_abc_inv_psm_2mods/afe_abc_inv_psm_mod1/inverter_control/current_ctrl/bemf_observer/phase_fault/double_integrator_observer/bounder1 ==
  data: u input; y output
function y = bounder(u)
    
    u = -pi + mod(u+3*pi,2*pi);
    
    y = u;
end

== matlab function afe_abc_inv_psm_2mods/afe_abc_inv_psm_mod1/afe_control/grid_voltage_phase_lock_loops/ddsrf_pll/pll_stageA/mormalization_and_transformation/abc2alphabeta ==
  data: a input; alpha output; b input; c input; beta output
function [alpha,beta] = abc2alphabeta(a,b,c)

alpha = 2/3*(a - 1/2*b - 1/2*c);
beta  = 1/sqrt(3)*(b - c);

end

== matlab function afe_abc_inv_psm_2mods/afe_abc_inv_psm_mod1/afe_control/grid_voltage_phase_lock_loops/ddsrf_pll/pll_stageA/sequences/ddsrf/alphabeta2xieta_neg ==
  data: alpha input; xi output; beta input; gamma input; eta output
function [xi,eta] = alphabeta2xieta_neg(alpha,beta,gamma)

    xi  = alpha*cos(gamma) - beta*sin(gamma);
    eta = alpha*sin(gamma) + beta*cos(gamma);

end

== matlab function afe_abc_inv_psm_2mods/afe_abc_inv_psm_mod1/afe_control/grid_voltage_phase_lock_loops/ddsrf_pll/pll_stageA/sequences/ddsrf/alphabeta2xieta_neg1 ==
  data: alpha input; xi output; beta input; gamma input; eta output
function [xi,eta] = alphabeta2xieta_neg(alpha,beta,gamma)

    xi  = alpha*cos(gamma) - beta*sin(gamma);
    eta = alpha*sin(gamma) + beta*cos(gamma);

end

== matlab function afe_abc_inv_psm_2mods/afe_abc_inv_psm_mod1/afe_control/grid_voltage_phase_lock_loops/ddsrf_pll/pll_stageA/sequences/ddsrf/alphabeta2xieta_pos ==
  data: alpha input; xi output; beta input; gamma input; eta output
function [xi,eta] = alphabeta2xieta_pos(alpha,beta,gamma)

    xi  =  alpha*cos(gamma) + beta*sin(gamma);
    eta = -alpha*sin(gamma) + beta*cos(gamma);

end

== matlab function afe_abc_inv_psm_2mods/afe_abc_inv_psm_mod1/afe_control/grid_voltage_phase_lock_loops/ddsrf_pll/pll_stageA/sequences/ddsrf/alphabeta2xieta_pos1 ==
  data: alpha input; xi output; beta input; gamma input; eta output
function [xi,eta] = alphabeta2xieta_pos(alpha,beta,gamma)

    xi  =  alpha*cos(gamma) + beta*sin(gamma);
    eta = -alpha*sin(gamma) + beta*cos(gamma);

end

== matlab function afe_abc_inv_psm_2mods/afe_abc_inv_psm_mod1/afe_control/grid_voltage_phase_lock_loops/ddsrf_pll/pll_stageA/sequences/ddsrf/bounder2 ==
  data: u input; y output
function y = bounder(u)
    
    y = -pi + mod(u+3*pi,2*pi);
    
end

== matlab function afe_abc_inv_psm_2mods/afe_abc_inv_psm_mod1/afe_control/grid_voltage_phase_lock_loops/ddsrf_pll/pll_stageB/bounder1 ==
  data: u input; y output
function y = bounder(u)
    y = -pi + mod(u+3*pi,2*pi);
end

== matlab function afe_abc_inv_psm_2mods/afe_abc_inv_psm_mod1/afe_control/grid_voltage_phase_lock_loops/ddsrf_pll/pll_stageB/double_integrator_observer/bounder1 ==
  data: u input; y output
function y = bounder(u)
    
    y = -pi + mod(u+3*pi,2*pi);
    
end

== matlab function afe_abc_inv_psm_2mods/grid/grid_emulator/grid_emulator/voltage_reference/alphabeta2abc ==
  data: alpha input; a output; beta input; b output; c output
function [a,b,c] = alphabeta2abc(alpha,beta)

    a  =  alpha;
    b  =  -0.5*alpha + sqrt(3)/2*beta;
    c  =  -0.5*alpha - sqrt(3)/2*beta;
end

== matlab function afe_abc_inv_psm_2mods/afe_abc_inv_psm_mod1/afe_control/grid_voltage_phase_lock_loops/ddsrf_pll/pll_stageB/double_integrator_observer/bounder2 ==
  data: u input; y output
function y = bounder(u)
    
    y = -pi + mod(u+3*pi,2*pi);
    
end

== matlab function afe_abc_inv_psm_2mods/afe_abc_inv_psm_mod2/afe/sv_pwm/modulator1/PWM generator 1/MATLAB Function ==
  data: t input; y output; phase input; period input
function y = trgo(t,phase,period)
x = sin(2*pi/period*t - phase -pi/2);
y = asin(x);

== matlab function afe_abc_inv_psm_2mods/afe_abc_inv_psm_mod2/afe/sv_pwm/modulator1/PWM generator 2/MATLAB Function ==
  data: t input; y output; phase input; period input
function y = trgo(t,phase,period)
x = sin(2*pi/period*t - phase -pi/2);
y = asin(x);

== matlab function afe_abc_inv_psm_2mods/afe_abc_inv_psm_mod2/afe/sv_pwm/modulator1/PWM generator 3/MATLAB Function ==
  data: t input; y output; phase input; period input
function y = trgo(t,phase,period)
x = sin(2*pi/period*t - phase -pi/2);
y = asin(x);

== matlab function afe_abc_inv_psm_2mods/afe_abc_inv_psm_mod2/afe_control/current_ctrl/Inner Loop Current Control/MATLAB Function ==
  data: a input; alpha output; b input; c input; beta output
function [alpha,beta] = abc2alphabeta(a,b,c)

alpha = 2/3*(a - 1/2*b - 1/2*c);
beta  = 1/sqrt(3)*(b - c);

end

== matlab function afe_abc_inv_psm_2mods/afe_abc_inv_psm_mod2/afe_control/current_ctrl/current_transformation/alphabeta2xieta ==
  data: alpha input; xi output; beta input; gamma input; eta output
function [xi,eta] = alphabeta2xieta(alpha,beta,gamma)

    xi  =  alpha*cos(gamma) + beta*sin(gamma);
    eta = -alpha*sin(gamma) + beta*cos(gamma);

end

== matlab function afe_abc_inv_psm_2mods/afe_abc_inv_psm_mod2/afe_control/current_ctrl/current_transformation/uvw2alphabeta ==
  data: u input; alpha output; v input; w input; beta output
function [alpha,beta] = uvw2alphabeta(u,v,w)

alpha = 2/3*(u - 1/2*v - 1/2*w);
beta  = 2/3*(sqrt(3)/2*(v - w));

end

== matlab function afe_abc_inv_psm_2mods/afe_abc_inv_psm_mod2/afe_control/current_ctrl/xieta2abc/MATLAB Function2 ==
  data: alpha input; a output; beta input; b output; c output
function [a,b,c] = alphabeta2abc(alpha,beta)

a = alpha;
b = -(1/2)*alpha + sqrt(3)/2*beta;
c = -(1/2)*alpha - sqrt(3)/2*beta;

end

== matlab function afe_abc_inv_psm_2mods/afe_abc_inv_psm_mod2/afe_control/current_ctrl/xieta2abc/Negative Sequence ==
  data: xi input; alpha output; eta input; gamma input; beta output
function [alpha,beta] = neg2alphabeta(xi,eta,gamma)

    alpha = xi*cos(gamma)  + eta*sin(gamma);
    beta  = -xi*sin(gamma) + eta*cos(gamma);

end

== matlab function afe_abc_inv_psm_2mods/afe_abc_inv_psm_mod2/afe_control/current_ctrl/xieta2abc/Positive Sequence ==
  data: xi input; alpha output; eta input; gamma input; beta output
function [alpha,beta] = pos2alphabeta(xi,eta,gamma)

    alpha = xi*cos(gamma) - eta*sin(gamma);
    beta  = xi*sin(gamma) + eta*cos(gamma);

end

== matlab function afe_abc_inv_psm_2mods/afe_abc_inv_psm_mod2/afe_control/grid_current_sampling_and_alpha_beta_transformation/i_abc2alphabeta ==
  data: i_abc input; alpha output; beta output
function [alpha,beta] = abc2alphabeta(i_abc)

alpha = 2/3*(i_abc(1) - 1/2*i_abc(2) - 1/2*i_abc(3));
beta  = 1/sqrt(3)*(i_abc(2) - i_abc(3));

end

== matlab function afe_abc_inv_psm_2mods/grid/grid_emulator/grid_emulator/voltage_reference/xieta2alphabeta_neg ==
  data: xi input; alpha output; eta input; gamma input; beta output
function [alpha,beta] = xieta2alphabeta_neg(xi,eta,gamma)

    alpha  =  xi*cos(gamma) + eta*sin(gamma);
    beta = -xi*sin(gamma) + eta*cos(gamma);

end

== matlab function afe_abc_inv_psm_2mods/afe_abc_inv_psm_mod2/afe_control/grid_voltage_phase_lock_loops/DDSRF-PLL/pll_stageA/mormalization_and_transformation/abc2alphabeta ==
  data: a input; alpha output; b input; c input; beta output
function [alpha,beta] = abc2alphabeta(a,b,c)

alpha = 2/3*(a - 1/2*b - 1/2*c);
beta  = 1/sqrt(3)*(b - c);

end

== matlab function afe_abc_inv_psm_2mods/afe_abc_inv_psm_mod2/afe_control/grid_voltage_phase_lock_loops/DDSRF-PLL/pll_stageA/sequences/ddsrf/alphabeta2xieta_neg ==
  data: alpha input; xi output; beta input; gamma input; eta output
function [xi,eta] = alphabeta2xieta_neg(alpha,beta,gamma)

    xi  = alpha*cos(gamma) - beta*sin(gamma);
    eta = alpha*sin(gamma) + beta*cos(gamma);

end

== matlab function afe_abc_inv_psm_2mods/afe_abc_inv_psm_mod2/afe_control/grid_voltage_phase_lock_loops/DDSRF-PLL/pll_stageA/sequences/ddsrf/alphabeta2xieta_neg1 ==
  data: alpha input; xi output; beta input; gamma input; eta output
function [xi,eta] = alphabeta2xieta_neg(alpha,beta,gamma)

    xi  = alpha*cos(gamma) - beta*sin(gamma);
    eta = alpha*sin(gamma) + beta*cos(gamma);

end

== matlab function afe_abc_inv_psm_2mods/afe_abc_inv_psm_mod2/afe_control/grid_voltage_phase_lock_loops/DDSRF-PLL/pll_stageA/sequences/ddsrf/alphabeta2xieta_pos ==
  data: alpha input; xi output; beta input; gamma input; eta output
function [xi,eta] = alphabeta2xieta_pos(alpha,beta,gamma)

    xi  =  alpha*cos(gamma) + beta*sin(gamma);
    eta = -alpha*sin(gamma) + beta*cos(gamma);

end

== matlab function afe_abc_inv_psm_2mods/afe_abc_inv_psm_mod2/afe_control/grid_voltage_phase_lock_loops/DDSRF-PLL/pll_stageA/sequences/ddsrf/alphabeta2xieta_pos1 ==
  data: alpha input; xi output; beta input; gamma input; eta output
function [xi,eta] = alphabeta2xieta_pos(alpha,beta,gamma)

    xi  =  alpha*cos(gamma) + beta*sin(gamma);
    eta = -alpha*sin(gamma) + beta*cos(gamma);

end

== matlab function afe_abc_inv_psm_2mods/afe_abc_inv_psm_mod2/afe_control/grid_voltage_phase_lock_loops/DDSRF-PLL/pll_stageA/sequences/ddsrf/bounder2 ==
  data: u input; y output
function y = bounder(u)
    
    y = -pi + mod(u+3*pi,2*pi);
    
end

== matlab function afe_abc_inv_psm_2mods/afe_abc_inv_psm_mod2/afe_control/grid_voltage_phase_lock_loops/DDSRF-PLL/pll_stageB/bounder1 ==
  data: u input; y output
function y = bounder(u)
    y = -pi + mod(u+3*pi,2*pi);
end

== matlab function afe_abc_inv_psm_2mods/afe_abc_inv_psm_mod2/afe_control/grid_voltage_phase_lock_loops/DDSRF-PLL/pll_stageB/double_integrator_observer/bounder1 ==
  data: u input; y output
function y = bounder(u)
    
    y = -pi + mod(u+3*pi,2*pi);
    
end

== matlab function afe_abc_inv_psm_2mods/afe_abc_inv_psm_mod2/afe_control/grid_voltage_phase_lock_loops/DDSRF-PLL/pll_stageB/double_integrator_observer/bounder2 ==
  data: u input; y output
function y = bounder(u)
    
    y = -pi + mod(u+3*pi,2*pi);
    
end

== matlab function afe_abc_inv_psm_2mods/afe_abc_inv_psm_mod2/afe_control/grid_voltage_phase_lock_loops/DQ-PLL/pll_stageA/mormalization_and_transformation/abc2alphabeta ==
  data: a input; alpha output; b input; c input; beta output
function [alpha,beta] = abc2alphabeta(a,b,c)

alpha = 2/3*(a - 1/2*b - 1/2*c);
beta  = 1/sqrt(3)*(b - c);

end
